simulink model "monosyn_multiscale"  (Simulink 7.8)
settings: Solver=ode2  StartTime=0.0  StopTime=15  FixedStep=T  RelTol=1e-3
InitFcn:
  | [A tau T] = emg_filter();
  | up = generate_min_jerk( 1, 1.1, 1.5, T );
  | down = 2.1 - up;
  | stretch = [repmat([up; down], 2, 1); [up ;down]];
  | l = length(stretch);
  | stretch(1 : ceil(l/3), 2) = 1;
  | stretch(:, 1) = [0:l-1]*T;
  | 
  | for i = 1:20
  |     eval(['SIZE_MU_', num2str(i), '=', num2str('(atan(150) - atan(i^0.8)) * 6;')])
  | end
StopFcn:
  | %recruitment_pattern_plotter(spikes_g1, spikes_g2, total_force, 0.02)
  | %incrementVars('emg_spasticity')
values from neighbouring files (symbols this model uses):
  A = exp(-T/tau)    [emg_filter.m]
  T = 1/1024    (= 0.0009765625)    [emg_filter.m]    (also in get_active_function_coeff.m; set_trfcn.m = 0.001)
  tau = 0.03    [emg_filter.m]
undefined symbols (not defined in the file or in its folder): dfilt, fdesignblkfcn, gcbh, SIZE_MU_1, SIZE_MU_10, SIZE_MU_11, SIZE_MU_12, SIZE_MU_13, SIZE_MU_14, SIZE_MU_15, SIZE_MU_16, SIZE_MU_17, SIZE_MU_18, SIZE_MU_19, SIZE_MU_2, SIZE_MU_20, SIZE_MU_3, SIZE_MU_4, SIZE_MU_5, SIZE_MU_6, SIZE_MU_7, SIZE_MU_8, SIZE_MU_9
libraries: simulink x4, cstblocks x1, dsparch4 x1
settings Model: Creator=minos_niu  LastModifiedBy=minos_niu

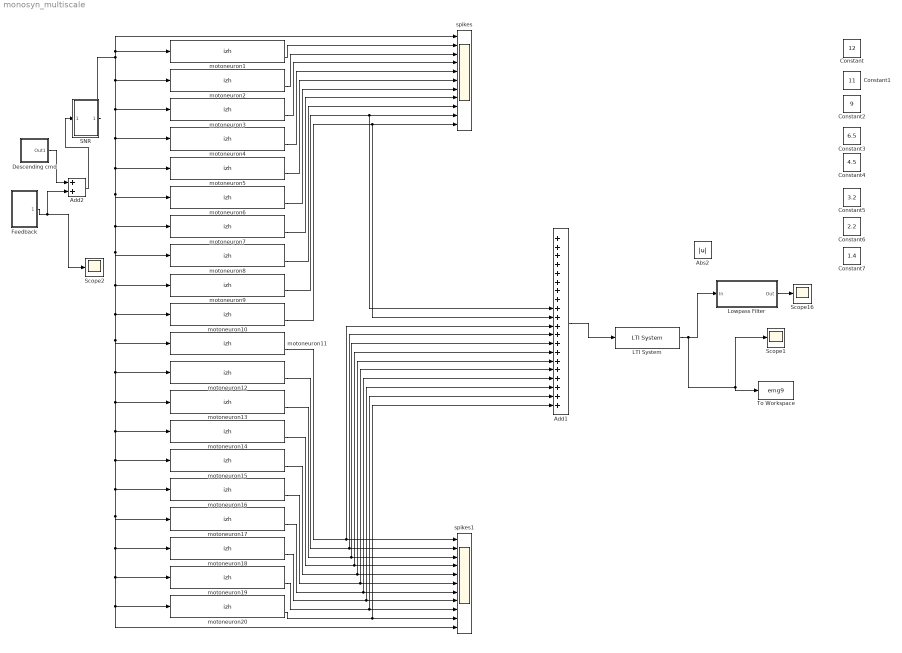
== system monosyn_multiscale ==
  Abs2 : Abs
  Add1 : Sum  Inputs=++++++++++++++++++++
  Add2 : Sum
  Constant : Constant  Value=12
  Constant1 : Constant  Value=11
  Constant2 : Constant  Value=9
  Constant3 : Constant  Value=6.5
  Constant4 : Constant  Value=4.5
  Constant5 : Constant  Value=3.2
  Constant6 : Constant  Value=2.2
  Constant7 : Constant  Value=1.4
  Descending cmd : Subsystem
  Feedback : Subsystem
  LTI System : cstblocks/LTI System  sys=zpk([0], [A A], 2*T*A, T) - zpk([0 -A], [A A A], T^2*A/tau, T)  IC=[]
  Lowpass Filter : Subsystem  DialogController=fdesignblkfcn  DialogControllerArgs=DataTag1  InitFcn=fdesignblkfcn(gcbh, {'InitFcn'});
      settings: CopyFcn=fdesignblkfcn(gcbh, {'CopyFcn'});
      mask Type: Lowpass Filter
      mask Description: Design a lowpass filter
      mask Help: helpview(mapfilelocation('dsp'), 'dsplowpassfilter');
      mask Display: disp('Lowpass')
  SNR : Subsystem
  Scope1 : Scope
      settings: YMin=0  YMax=450000  SaveName=ScopeData2
  Scope16 : Scope
      settings: TimeRange=10  YMin=0  YMax=350000  SaveName=total_force  DataFormat=Structure
  Scope2 : Scope
      settings: TimeRange=10  YMin=0  YMax=350000  SaveName=total_force1  DataFormat=Structure
  To Workspace : ToWorkspace  VariableName=emg9  SampleTime=-1  SaveFormat=Structure With Time
  motoneuron1 : S-Function  FunctionName=izh  Parameters=[0.02 0.2 -65.0 6.0 30.0 SIZE_MU_1] [-70.0 -14.0]  EnableBusSupport=off
      mask Display:
      | port_label('input', 1, 'syn curr');
      | port_label('output', 1, 'action potential');
      | port_label('output', 2, 'spike');
      | disp('Izhi Neuron \n(S-Function)')
  motoneuron10 : S-Function  FunctionName=izh  Parameters=[0.02 0.2 -65.0 6.0 30.0 SIZE_MU_10] [-70.0 -14.0]  EnableBusSupport=off
      mask Display:
      | port_label('input', 1, 'syn curr');
      | port_label('output', 1, 'action potential');
      | port_label('output', 2, 'spike');
      | disp('Izhi Neuron \n(S-Function)')
  motoneuron11 : S-Function  FunctionName=izh  Parameters=[0.02 0.2 -65.0 6.0 30.0 SIZE_MU_11] [-70.0 -14.0]  EnableBusSupport=off
      mask Display:
      | port_label('input', 1, 'syn curr');
      | port_label('output', 1, 'action potential');
      | port_label('output', 2, 'spike');
      | disp('Izhi Neuron \n(S-Function)')
  motoneuron12 : S-Function  FunctionName=izh  Parameters=[0.02 0.2 -65.0 6.0 30.0 SIZE_MU_12] [-70.0 -14.0]  EnableBusSupport=off
      mask Display:
      | port_label('input', 1, 'syn curr');
      | port_label('output', 1, 'action potential');
      | port_label('output', 2, 'spike');
      | disp('Izhi Neuron \n(S-Function)')
  motoneuron13 : S-Function  FunctionName=izh  Parameters=[0.02 0.2 -65.0 6.0 30.0 SIZE_MU_13] [-70.0 -14.0]  EnableBusSupport=off
      mask Display:
      | port_label('input', 1, 'syn curr');
      | port_label('output', 1, 'action potential');
      | port_label('output', 2, 'spike');
      | disp('Izhi Neuron \n(S-Function)')
  motoneuron14 : S-Function  FunctionName=izh  Parameters=[0.02 0.2 -65.0 6.0 30.0 SIZE_MU_14] [-70.0 -14.0]  EnableBusSupport=off
      mask Display:
      | port_label('input', 1, 'syn curr');
      | port_label('output', 1, 'action potential');
      | port_label('output', 2, 'spike');
      | disp('Izhi Neuron \n(S-Function)')
  motoneuron15 : S-Function  FunctionName=izh  Parameters=[0.02 0.2 -65.0 6.0 30.0 SIZE_MU_15] [-70.0 -14.0]  EnableBusSupport=off
      mask Display:
      | port_label('input', 1, 'syn curr');
      | port_label('output', 1, 'action potential');
      | port_label('output', 2, 'spike');
      | disp('Izhi Neuron \n(S-Function)')
  motoneuron16 : S-Function  FunctionName=izh  Parameters=[0.02 0.2 -65.0 6.0 30.0 SIZE_MU_16] [-70.0 -14.0]  EnableBusSupport=off
      mask Display:
      | port_label('input', 1, 'syn curr');
      | port_label('output', 1, 'action potential');
      | port_label('output', 2, 'spike');
      | disp('Izhi Neuron \n(S-Function)')
  motoneuron17 : S-Function  FunctionName=izh  Parameters=[0.02 0.2 -65.0 6.0 30.0 SIZE_MU_17] [-70.0 -14.0]  EnableBusSupport=off
      mask Display:
      | port_label('input', 1, 'syn curr');
      | port_label('output', 1, 'action potential');
      | port_label('output', 2, 'spike');
      | disp('Izhi Neuron \n(S-Function)')
  motoneuron18 : S-Function  FunctionName=izh  Parameters=[0.02 0.2 -65.0 6.0 30.0 SIZE_MU_18] [-70.0 -14.0]  EnableBusSupport=off
      mask Display:
      | port_label('input', 1, 'syn curr');
      | port_label('output', 1, 'action potential');
      | port_label('output', 2, 'spike');
      | disp('Izhi Neuron \n(S-Function)')
  motoneuron19 : S-Function  FunctionName=izh  Parameters=[0.02 0.2 -65.0 6.0 30.0 SIZE_MU_19] [-70.0 -14.0]  EnableBusSupport=off
      mask Display:
      | port_label('input', 1, 'syn curr');
      | port_label('output', 1, 'action potential');
      | port_label('output', 2, 'spike');
      | disp('Izhi Neuron \n(S-Function)')
  motoneuron2 : S-Function  FunctionName=izh  Parameters=[0.02 0.2 -65.0 6.0 30.0 SIZE_MU_2] [-70.0 -14.0]  EnableBusSupport=off
      mask Display:
      | port_label('input', 1, 'syn curr');
      | port_label('output', 1, 'action potential');
      | port_label('output', 2, 'spike');
      | disp('Izhi Neuron \n(S-Function)')
  motoneuron20 : S-Function  FunctionName=izh  Parameters=[0.02 0.2 -65.0 6.0 30.0 SIZE_MU_20] [-70.0 -14.0]  EnableBusSupport=off
      mask Display:
      | port_label('input', 1, 'syn curr');
      | port_label('output', 1, 'action potential');
      | port_label('output', 2, 'spike');
      | disp('Izhi Neuron \n(S-Function)')
  motoneuron3 : S-Function  FunctionName=izh  Parameters=[0.02 0.2 -65.0 6.0 30.0 SIZE_MU_3] [-70.0 -14.0]  EnableBusSupport=off
      mask Display:
      | port_label('input', 1, 'syn curr');
      | port_label('output', 1, 'action potential');
      | port_label('output', 2, 'spike');
      | disp('Izhi Neuron \n(S-Function)')
  motoneuron4 : S-Function  FunctionName=izh  Parameters=[0.02 0.2 -65.0 6.0 30.0 SIZE_MU_4] [-70.0 -14.0]  EnableBusSupport=off
      mask Display:
      | port_label('input', 1, 'syn curr');
      | port_label('output', 1, 'action potential');
      | port_label('output', 2, 'spike');
      | disp('Izhi Neuron \n(S-Function)')
  motoneuron5 : S-Function  FunctionName=izh  Parameters=[0.02 0.2 -65.0 6.0 30.0 SIZE_MU_5] [-70.0 -14.0]  EnableBusSupport=off
      mask Display:
      | port_label('input', 1, 'syn curr');
      | port_label('output', 1, 'action potential');
      | port_label('output', 2, 'spike');
      | disp('Izhi Neuron \n(S-Function)')
  motoneuron6 : S-Function  FunctionName=izh  Parameters=[0.02 0.2 -65.0 6.0 30.0 SIZE_MU_6] [-70.0 -14.0]  EnableBusSupport=off
      mask Display:
      | port_label('input', 1, 'syn curr');
      | port_label('output', 1, 'action potential');
      | port_label('output', 2, 'spike');
      | disp('Izhi Neuron \n(S-Function)')
  motoneuron7 : S-Function  FunctionName=izh  Parameters=[0.02 0.2 -65.0 6.0 30.0 SIZE_MU_7] [-70.0 -14.0]  EnableBusSupport=off
      mask Display:
      | port_label('input', 1, 'syn curr');
      | port_label('output', 1, 'action potential');
      | port_label('output', 2, 'spike');
      | disp('Izhi Neuron \n(S-Function)')
  motoneuron8 : S-Function  FunctionName=izh  Parameters=[0.02 0.2 -65.0 6.0 30.0 SIZE_MU_8] [-70.0 -14.0]  EnableBusSupport=off
      mask Display:
      | port_label('input', 1, 'syn curr');
      | port_label('output', 1, 'action potential');
      | port_label('output', 2, 'spike');
      | disp('Izhi Neuron \n(S-Function)')
  motoneuron9 : S-Function  FunctionName=izh  Parameters=[0.02 0.2 -65.0 6.0 30.0 SIZE_MU_9] [-70.0 -14.0]  EnableBusSupport=off
      mask Display:
      | port_label('input', 1, 'syn curr');
      | port_label('output', 1, 'action potential');
      | port_label('output', 2, 'spike');
      | disp('Izhi Neuron \n(S-Function)')
  spikes : Scope  NumInputPorts=11
      settings: TickLabels=on  TimeRange=5  YMin=-1000~-5~-5~-5~-5~-5~-5~-5~-5~-5~-5  YMax=5000~5~5~5~5~5~5~5~5~5~5  SaveName=spikes_g1  DataFormat=Structure
  spikes1 : Scope  NumInputPorts=11
      settings: TickLabels=on  TimeRange=5  YMin=0~-1~-1~-1~-1~-1~-1~-1~-1~-1~1.25  YMax=12500~1~1~1~1~1~1~1~1~1~4  SaveName=spikes_g2  DataFormat=Structure
  wires:
  motoneuron1/2 -> spikes/2
  Lowpass Filter/1(Out) -> Scope16/1
  motoneuron2/2 -> spikes/3
  motoneuron3/2 -> spikes/4
  motoneuron4/2 -> spikes/5
  motoneuron5/2 -> spikes/6
  motoneuron6/2 -> spikes/7
  motoneuron7/2 -> spikes/8
  motoneuron9/2 -> spikes/10, Add1/9
  LTI System/1 -> Lowpass Filter/1(In), Scope1/1, To Workspace/1
  motoneuron20/2 -> spikes1/10, Add1/20
  motoneuron19/2 -> spikes1/9, Add1/19
  motoneuron18/2 -> spikes1/8, Add1/18
  motoneuron17/2 -> spikes1/7, Add1/17
  motoneuron16/2 -> spikes1/6, Add1/16
  motoneuron15/2 -> spikes1/5, Add1/15
  motoneuron14/2 -> spikes1/4, Add1/14
  motoneuron13/2 -> spikes1/3, Add1/13
  motoneuron12/2 -> spikes1/2, Add1/12
  motoneuron11/2 -> spikes1/1, Add1/11
  motoneuron10/2 -> spikes/11, Add1/10
  Add1/1 -> LTI System/1
  motoneuron8/2 -> spikes/9
  Descending cmd/1(Out1) -> Add2/1
  SNR/1(Out1) -> spikes/1, motoneuron1/1, motoneuron2/1, motoneuron3/1, motoneuron4/1, motoneuron5/1, motoneuron6/1, motoneuron7/1, motoneuron8/1, motoneuron9/1, motoneuron10/1, motoneuron11/1, motoneuron12/1, motoneuron13/1, motoneuron14/1, motoneuron15/1, motoneuron16/1, motoneuron17/1, motoneuron18/1, motoneuron19/1, spikes1/11, motoneuron20/1
  Feedback/1(Ia_pps) -> Scope2/1, Add2/2
  Add2/1 -> SNR/1(In1)

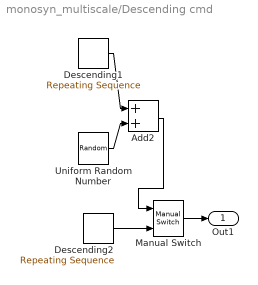
== system monosyn_multiscale/Descending cmd ==
  Add2 : Sum
  Descending1 : simulink/Sources/Repeating Sequence  rep_seq_t=[0 1.1 3.1 6.8 9.5 10 ]  rep_seq_y=[0 0 20 20 0 0]*1
  Descending2 : simulink/Sources/Repeating Sequence  rep_seq_t=[0 0.5 1]  rep_seq_y=[0 200 200]*0
  Manual Switch : simulink/Signal Routing/Manual Switch  sw=0  action=0  varsize=off
  Uniform Random Number : UniformRandomNumber  Minimum=-6  Maximum=0  SampleTime=T
  Out1 : Outport
  wires:
  Manual Switch/1 -> Out1/1
  Add2/1 -> Manual Switch/1
  Uniform Random Number/1 -> Add2/2
  Descending2/1 -> Manual Switch/2
  Descending1/1 -> Add2/1

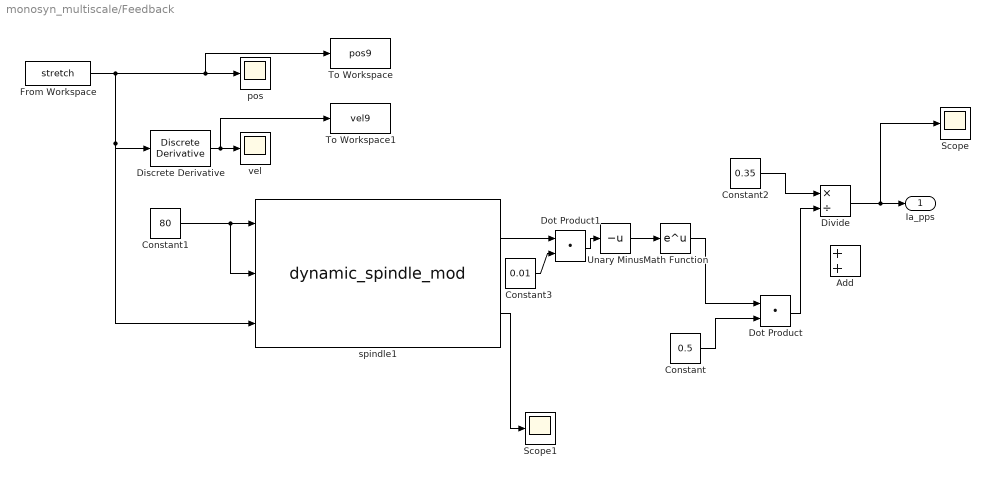
== system monosyn_multiscale/Feedback ==
  Add : Sum
  Constant : Constant  Value=0.5
  Constant1 : Constant  Value=80
  Constant2 : Constant  Value=0.35
  Constant3 : Constant  Value=0.01
  Discrete Derivative : simulink/Discrete/Discrete Derivative  gainval=1.0  ICPrevScaledInput=0  InputProcessing=Inherited  OutMin=[]  OutMax=[]  OutDataType=fixdt(1, 16)  OutScaling=2^-10  DoSatur=off
  Divide : Product  Inputs=*/
  Dot Product : DotProduct  InputSameDT=on  OutDataTypeStr=Inherit: Inherit via internal rule
  Dot Product1 : DotProduct  InputSameDT=on  OutDataTypeStr=Inherit: Inherit via internal rule
  From Workspace : FromWorkspace  VariableName=stretch  SampleTime=T
  Math Function : Math  SaturateOnIntegerOverflow=on
  Scope : Scope
      settings: YMin=0  YMax=225
  Scope1 : Scope
      settings: TimeRange=1  SaveName=ScopeData4
  To Workspace : ToWorkspace  VariableName=pos9  SampleTime=-1  SaveFormat=Structure With Time
  To Workspace1 : ToWorkspace  VariableName=vel9  SampleTime=-1  SaveFormat=Structure With Time
  Unary Minus : UnaryMinus
  pos : Scope
      settings: SaveName=ScopeData5
  spindle1 : S-Function  FunctionName=dynamic_spindle_mod  Parameters=[10.4649 10.4649 10.4649] [0.1127 0.1623 0.1623] [0.0605 0.0822 0.0822] [0.2356 -0.046 -0.069] [0 0 0] [0.0289 0.0636 0.0954] [1 0.7 0.7] [1 0.92 0.92] [20000 10000 10000] [20000 7250 7250] [0.3 0.3 0.3] [0.46 0.46 0.46] [0.04 0.04 0.04] [0.76 0.76 0.76] [1 0.04 0.04] [0.192 0.185 0.0001] [0.0002 0.0002 0.0002] [1 0.5 1] [1]  EnableBusSupport=off
      mask Display:
      | port_label('input', 1, 'gamma dynamic');
      | port_label('input', 2, 'gamma static');
      | port_label('input', 3, 'Lce(L0)');
      | port_label('output',1,'Ia');
      | port_label('output',2,'II');
      | disp('Muscle Spindle \n(S-Function)')
  vel : Scope
      settings: SaveName=ScopeData6
  Ia_pps : Outport
  wires:
  From Workspace/1 -> Discrete Derivative/1, spindle1/3, pos/1, To Workspace/1
  Discrete Derivative/1 -> vel/1, To Workspace1/1
  Constant1/1 -> spindle1/2, spindle1/1
  spindle1/1 -> Dot Product1/1
  spindle1/2 -> Scope1/1
  Math Function/1 -> Dot Product/1
  Constant/1 -> Dot Product/2
  Unary Minus/1 -> Math Function/1
  Constant2/1 -> Divide/1
  Dot Product/1 -> Divide/2
  Divide/1 -> Ia_pps/1, Scope/1
  Constant3/1 -> Dot Product1/2
  Dot Product1/1 -> Unary Minus/1

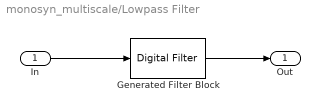
== system monosyn_multiscale/Lowpass Filter ==
  In : Inport
  Generated Filter Block : dsparch4/Digital Filter  Tag=BlockMethodSubSystem  TypePopup=FIR (all zeros)  IIRFiltStruct=Direct form II transposed  AllPoleFiltStruct=Direct form  FIRFiltStruct=Direct form  CoeffSource=Specify via dialog  NumCoeffs=[0.000595204877442133 0.000254635190406011 0.000308047604271057 0.000367814132296875 0.000434478340747626 0.000508414988635158 0.000590035571175549 0.000679747654269358 0.000777868822071414 0.000884633472779032 0.00100035572983715 0.00112521614601972 0.00125966125920154 0.0014038444034124 0.00155818955783148 0.00172274011508705 0.00189770797205443 0.00208297564909501 0.0022786519245691 0.00248478477740101 0.00270160686757103 0.0029289827639676 0.00316674641779681 0.00341421414193548 0.0036716702932362 0.00393883449431907 0.00421601466996312 0.00450114503951654 0.00479506915687342 0.00509786388878379 0.00540724274319257 0.00572444915888108 0.00604746789391836 0.0063765201295102 0.00671030230122185 0.0070484824019172 0.0073899679144478 0.00773419237306669 0.00808006255844603 0.00842683992849057 0.00877340925258363 0.00911908480028514 0.00946269988278409 0.00980346170608762 0.0101400793790188 0.0104717895372354 0.0107974608415816 0.0111162571259452 0.0114270021557036 0.011728643698953 0.0120203518540101 0.0123012080166268 0.0125702299285631 0.0128265052480324 0.0130690191377833 0.0132974506299961 0.0135103210655435 0.0137075043052072 0.0138879656016236 0.0140512054144866 0.0141967056926303 0.01432377942794 0.0144321325450738 0.0145213248308461 0.014591073590015 0.0146410580526161 0.0146710664886973 0.0146810925552542 0.0146710664886973 0.0146410580526161 0.014591073590015 0.0145213248308461 0.0144321325450738 0.01432377942794 0.0141967056926303 0.0140512054144866 0.0138879656016236 0.0137075043052072 0.0135103210655435 0.0132974506299961 0.0130690191377833 0.0128265052480324 0.0125702299285631 0.0123012080166268 0.0120203518540101 0.011728643698953 0.0114270021557036 0.0111162571259452 0.0107974608415816 0.0104717895372354 0.0101400793790188 0.00980346170608762 0.00946269988278409 0.00911908480028514 0.00877340925258363 0.00842683992849057 0.00808006255844603 0.00773419237306669 0.0073899679144478 0.0070484824019172 0.00671030230122185 0.0063765201295102 0.00604746789391836 0.00572444915888108 0.00540724274319257 0.00509786388878379 0.00479506915687342 0.00450114503951654 0.00421601466996312 0.00393883449431907 0.0036716702932362 0.00341421414193548 0.00316674641779681 0.0029289827639676 0.00270160686757103 0.00248478477740101 0.0022786519245691 0.00208297564909501 0.00189770797205443 0.00172274011508705 0.00155818955783148 0.0014038444034124 0.00125966125920154 0.00112521614601972 0.00100035572983715 0.000884633472779032 0.000777868822071414 0.000679747654269358 0.000590035571175549 0.000508414988635158 0.000434478340747626 0.000367814132296875 0.000308047604271057 0.000254635190406011 0.000595204877442133]  DenCoeffs=[1 0.1]  BiQuadCoeffs=[1 0.3 0.4 1 0.1 0.2]  LatticeCoeffs=[0.2 0.4]  denIgnore=on  FiltPerSampPopup=One filter per frame  IC=0  ICnum=0  ICden=0  roundingMode=Floor  overflowMode=off  ScaleValues=1  scaleValueFracLength=14  stageInFracLength=15  stageOutFracLength=15  FilterSource=Specify via dialog  dfiltObjectName=dfilt.dffir([1 2 1])  InputProcessing=Columns as channels (frame based)
  Out : Outport
  wires:
  Generated Filter Block/1 -> Out/1
  In/1 -> Generated Filter Block/1

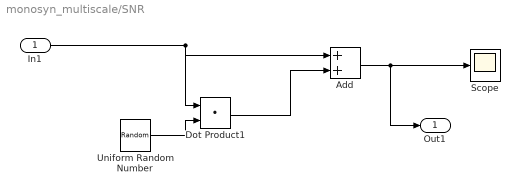
== system monosyn_multiscale/SNR ==
  In1 : Inport
  Add : Sum
  Dot Product1 : DotProduct  InputSameDT=on  OutDataTypeStr=Inherit: Inherit via internal rule
  Scope : Scope
  Uniform Random Number : UniformRandomNumber  Minimum=-0.3  Maximum=0.3  SampleTime=T
  Out1 : Outport
  wires:
  Uniform Random Number/1 -> Dot Product1/2
  In1/1 -> Dot Product1/1, Add/1
  Dot Product1/1 -> Add/2
  Add/1 -> Scope/1, Out1/1
